simulink model "anti_windup_DC_motor_discrete"  (R2021a)
settings: Solver=VariableStepAuto  StartTime=0.0  StopTime=200  RelTol=1e-3
libraries: pid_lib x2
settings Model: Creator=kjartan  LastModifiedBy=kjartan

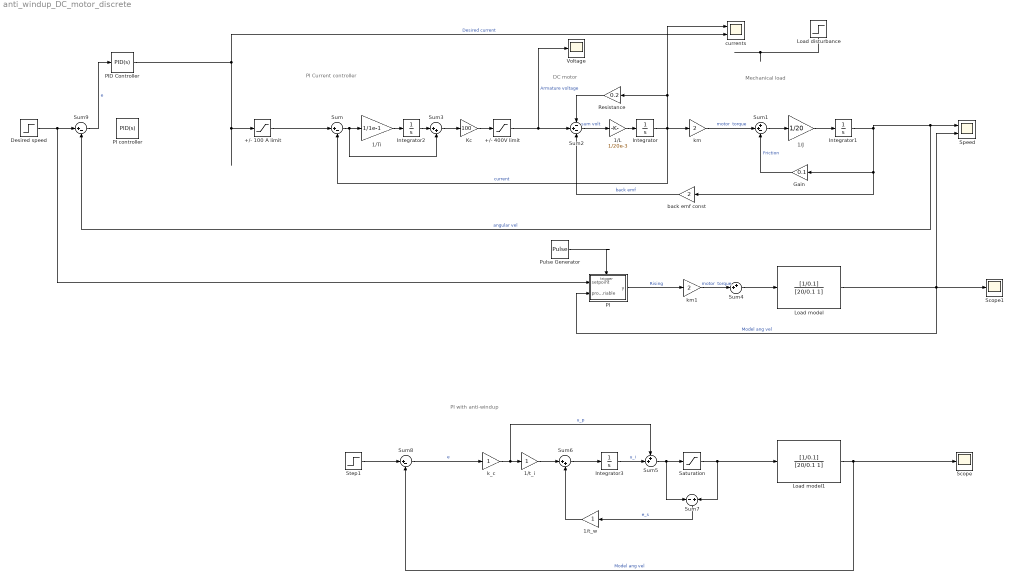
== system anti_windup_DC_motor_discrete ==
  note: PI with anti-windup
  note: PI Current controller
  note: Mechanical load
  note: DC motor
  +/- 100 A limit : Saturate  UpperLimit=100  LowerLimit=-100
  +/- 400V limit : Saturate  UpperLimit=400  LowerLimit=-400
  1/J : Gain  Gain=1/20
  1/L : Gain  Gain=1/20e-3
  1/Ti : Gain  Gain=1/1e-1
  1/t_i : Gain
  1/t_w : Gain
  Desired speed : Step  Time=0  After=100  SampleTime=0
  Gain : Gain  Gain=0.1
  Integrator{,1..3} (4 alike) : Integrator
  Kc : Gain  Gain=100
  Load disturbance : Step  Time=10  After=10  SampleTime=0
  Load model : TransferFcn  Numerator=[1/0.1]  Denominator=[20/0.1 1]
  Load model1 : TransferFcn  Numerator=[1/0.1]  Denominator=[20/0.1 1]
  PI : Subsystem
  PI controller : pid_lib/PID Controller  Controller=PID  Form=Ideal  TimeDomain=Continuous-time  UseExternalTs=off  SampleTime=-1  IntegratorMethod=Forward Euler  FilterMethod=Forward Euler  ControllerParametersSource=internal  P=10  I=1/20  D=20  UseFilter=on  N=100  TunerSelectOption=Transfer Function Based (PID Tuner App)  InitialConditionSource=internal  InitialConditionForIntegrator=0  InitialConditionForFilter=0  DifferentiatorICPrevScaledInput=0  ExternalReset=none  TrackingMode=off  Kt=1  LimitOutput=off  SatLimitsSource=internal  UpperSaturationLimit=inf  LowerSaturationLimit=-inf  LinearizeAsGain=on  AntiWindupMode=none  Kb=1  POutMin=[]  POutMax=[]  IOutMin=[]  IOutMax=[]  DOutMin=[]  DOutMax=[]  NOutMin=[]  NOutMax=[]  SumOutMin=[]  SumOutMax=[]  SaturationOutMin=[]  SaturationOutMax=[]  PParamMin=[]  PParamMax=[]  IParamMin=[]  IParamMax=[]  DParamMin=[]  DParamMax=[]  NParamMin=[]  NParamMax=[]  KbParamMin=[]  KbParamMax=[]  KtParamMin=[]  KtParamMax=[]  KbOutMin=[]  KbOutMax=[]  KtOutMin=[]  KtOutMax=[]  IntegratorOutMin=[]  IntegratorOutMax=[]  FilterOutMin=[]  FilterOutMax=[]  SumI1OutMin=[]  SumI1OutMax=[]  SumI2OutMin=[]  SumI2OutMax=[]  SumI3OutMin=[]  SumI3OutMax=[]  SumI4OutMin=[]  SumI4OutMax=[]  SumDOutMin=[]  SumDOutMax=[]  DifferentiatorOutMin=[]  DifferentiatorOutMax=[]  FilterDiffOutCoefMin=[]  FilterDiffOutCoefMax=[]  ReciprocalOutMin=[]  ReciprocalOutMax=[]  SumDenOutMin=[]  SumDenOutMax=[]  SumNumOutMin=[]  SumNumOutMax=[]  DivideOutMin=[]  DivideOutMax=[]  UdiffTsProdOutMin=[]  UdiffTsProdOutMax=[]  NTsProdOutMin=[]  NTsProdOutMax=[]  UintegralTsProdOutMin=[]  UintegralTsProdOutMax=[]  UngainTsProdOutMin=[]  UngainTsProdOutMax=[]  IntegratorContinuousStateAttributes=''  IntegratorStateMustResolveToSignalObject=off  IntegratorRTWStateStorageClass=Auto  FilterContinuousStateAttributes=''  FilterStateMustResolveToSignalObject=off  FilterRTWStateStorageClass=Auto  ParallelPVariant=Passthrough  IdealPVariant=InternalParameters  IVariant=InternalParameters  DVariant=InternalParameters  IntegratorVariant=Continuous  SatVariant=Disabled  AWVariant=Passthrough  PCopyVariant=Disabled  TRVariant=Disabled  FdbkBlocksVariant=Forward  IdealPFdbkVariant=Disabled  SatFdbkVariant=Disabled  DerivativeFilterVariant=ContFilter  NVariant=InternalParameters  NCopyVariant=Disabled  FilterICVariant=InternalICsFilter  IntegratorICVariant=InternalICs  ExternalResetVariant=Disabled  TRSumVariant=Passthrough  SumFdbkVariant=Disabled  SumVariant=Sum_PID  TsampFilterVariant=InternalTs  TsampNgainVariant=Passthrough  TsampIntegralVariant=Passthrough  ExternalSaturationOutDataTypeStr=Inherit: Same as second input
  PID Controller : pid_lib/PID Controller  Controller=PID  Form=Ideal  TimeDomain=Continuous-time  UseExternalTs=off  SampleTime=-1  IntegratorMethod=Forward Euler  FilterMethod=Forward Euler  ControllerParametersSource=internal  P=20  I=1/2  D=0  UseFilter=on  N=100  TunerSelectOption=Transfer Function Based (PID Tuner App)  InitialConditionSource=internal  InitialConditionForIntegrator=0  InitialConditionForFilter=0  DifferentiatorICPrevScaledInput=0  ExternalReset=none  TrackingMode=off  Kt=1  LimitOutput=off  SatLimitsSource=internal  UpperSaturationLimit=inf  LowerSaturationLimit=-inf  LinearizeAsGain=on  AntiWindupMode=none  Kb=1  POutMin=[]  POutMax=[]  IOutMin=[]  IOutMax=[]  DOutMin=[]  DOutMax=[]  NOutMin=[]  NOutMax=[]  SumOutMin=[]  SumOutMax=[]  SaturationOutMin=[]  SaturationOutMax=[]  PParamMin=[]  PParamMax=[]  IParamMin=[]  IParamMax=[]  DParamMin=[]  DParamMax=[]  NParamMin=[]  NParamMax=[]  KbParamMin=[]  KbParamMax=[]  KtParamMin=[]  KtParamMax=[]  KbOutMin=[]  KbOutMax=[]  KtOutMin=[]  KtOutMax=[]  IntegratorOutMin=[]  IntegratorOutMax=[]  FilterOutMin=[]  FilterOutMax=[]  SumI1OutMin=[]  SumI1OutMax=[]  SumI2OutMin=[]  SumI2OutMax=[]  SumI3OutMin=[]  SumI3OutMax=[]  SumI4OutMin=[]  SumI4OutMax=[]  SumDOutMin=[]  SumDOutMax=[]  DifferentiatorOutMin=[]  DifferentiatorOutMax=[]  FilterDiffOutCoefMin=[]  FilterDiffOutCoefMax=[]  ReciprocalOutMin=[]  ReciprocalOutMax=[]  SumDenOutMin=[]  SumDenOutMax=[]  SumNumOutMin=[]  SumNumOutMax=[]  DivideOutMin=[]  DivideOutMax=[]  UdiffTsProdOutMin=[]  UdiffTsProdOutMax=[]  NTsProdOutMin=[]  NTsProdOutMax=[]  UintegralTsProdOutMin=[]  UintegralTsProdOutMax=[]  UngainTsProdOutMin=[]  UngainTsProdOutMax=[]  IntegratorContinuousStateAttributes=''  IntegratorStateMustResolveToSignalObject=off  IntegratorRTWStateStorageClass=Auto  FilterContinuousStateAttributes=''  FilterStateMustResolveToSignalObject=off  FilterRTWStateStorageClass=Auto  ParallelPVariant=Passthrough  IdealPVariant=InternalParameters  IVariant=InternalParameters  DVariant=InternalParameters  IntegratorVariant=Continuous  SatVariant=Disabled  AWVariant=Passthrough  PCopyVariant=Disabled  TRVariant=Disabled  FdbkBlocksVariant=Forward  IdealPFdbkVariant=Disabled  SatFdbkVariant=Disabled  DerivativeFilterVariant=ContFilter  NVariant=InternalParameters  NCopyVariant=Disabled  FilterICVariant=InternalICsFilter  IntegratorICVariant=InternalICs  ExternalResetVariant=Disabled  TRSumVariant=Passthrough  SumFdbkVariant=Disabled  SumVariant=Sum_PID  TsampFilterVariant=InternalTs  TsampNgainVariant=Passthrough  TsampIntegralVariant=Passthrough  ExternalSaturationOutDataTypeStr=Inherit: Same as second input
  Pulse Generator : DiscretePulseGenerator  PulseType=Time based  Period=1e-2  PulseWidth=5
  Resistance : Gain  Gain=0.2
  Saturation : Saturate
  Scope : Scope
  Scope1 : Scope
  Speed : Scope  NumInputPorts=2
  Step1 : Step  After=100  SampleTime=0
  Sum : Sum  Inputs=|+-
  Sum1 : Sum  Inputs=++-
  Sum2 : Sum  Inputs=-+-
  Sum3 : Sum  Inputs=|++
  Sum4 : Sum  Inputs=++|
  Sum5 : Sum  Inputs=++|
  Sum6 : Sum  Inputs=|++
  Sum7 : Sum  Inputs=-|+
  Sum8 : Sum  Inputs=|+-
  Sum9 : Sum  Inputs=|+-
  Voltage : Scope
  back emf const : Gain  Gain=2
  currents : Scope  NumInputPorts=2
  k_c : Gain
  km : Gain  Gain=2
  km1 : Gain  Gain=2
  wires:
  Integrator1/1 -> back emf const/1, Gain/1, Sum9/2, Speed/1  "angular vel"
  1/L/1 -> Integrator/1
  Integrator/1 -> Sum/2, currents/1, Resistance/1, km/1  "current"
  km/1 -> Sum1/2  "motor  torque"
  Sum1/1 -> 1/J/1
  1/J/1 -> Integrator1/1
  Gain/1 -> Sum1/3  "Friction"
  Sum2/1 -> 1/L/1  "sum volt"
  back emf const/1 -> Sum2/3  "back emf"
  +/- 400V limit/1 -> Voltage/1, Sum2/2  "Armature voltage"
  Resistance/1 -> Sum2/1
  Kc/1 -> +/- 400V limit/1
  Sum3/1 -> Kc/1
  Integrator2/1 -> Sum3/1
  1/Ti/1 -> Integrator2/1
  Sum/1 -> Sum3/2, 1/Ti/1
  +/- 100 A limit/1 -> Sum/1
  PID Controller/1 -> +/- 100 A limit/1, currents/2  "Desired current"
  Load disturbance/1 -> ?
  Sum4/1 -> Load model/1
  Load model/1 -> PI/2(process variable), Scope1/1, Speed/2  "Model ang vel"
  Sum5/1 -> Sum7/1, Saturation/1
  Saturation/1 -> Sum7/2, Load model1/1
  Integrator3/1 -> Sum5/2  "u_i"
  Sum6/1 -> Integrator3/1
  1/t_w/1 -> Sum6/2
  Sum7/1 -> 1/t_w/1  "e_s"
  Sum8/1 -> k_c/1  "e"
  Load model1/1 -> Scope/1, Sum8/2  "Model ang vel"
  1/t_i/1 -> Sum6/1
  k_c/1 -> Sum5/1, 1/t_i/1  "u_p"
  Step1/1 -> Sum8/1
  km1/1 -> Sum4/2  "motor  torque"
  Sum9/1 -> PID Controller/1  "e"
  Desired speed/1 -> PI/1(setpoint), Sum9/1
  Pulse Generator/1 -> PI/Trigger
  PI/1(y) -> km1/1  "Rising"

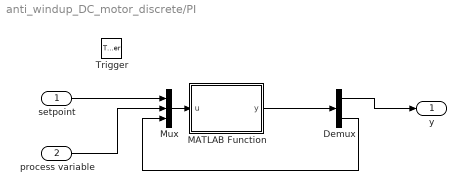
== system anti_windup_DC_motor_discrete/PI ==
  setpoint : Inport
  process variable : Inport  Port=2
  Trigger : TriggerPort  VariantControl=(inherit)
  Demux : Demux  Outputs=2
  MATLAB Function : MATLAB Function  TreatAsAtomicUnit=on
  Mux : Mux  Inputs=3
  y : Outport  InitialOutput=0  VectorParamsAs1DForOutWhenUnconnected=off
  wires:
  setpoint/1 -> Mux/1
  process variable/1 -> Mux/2
  Mux/1 -> MATLAB Function/1(u)
  MATLAB Function/1(y) -> Demux/1
  Demux/1 -> y/1
  Demux/2 -> Mux/3

== matlab function anti_windup_DC_motor_discrete/PI/MATLAB Function ==
  data: u input; y output
function y = PI_update(u)

% Anti-windup using backtracking

% Gains
kc = 10;
t_i = 2;
highlim = 100;
lowlim = -100;
h=0.01;

% Signals
sp = u(1); % Setpoint
pv = u(2); % process variable

uI = u(3); % Integral state

e = sp-pv; % Control error
v = kc*e + uI*kc/t_i;
if v > highlim
    y1 = highlim
    uI = uI - 1/t_i*(v-highlim);
elseif v < lowlim
    y1 = lowlim;
    uI = uI - 1/t_i*(v - lowlim);
else
    y1 = v;
    uI = uI + h*e;
end
y = [y1;uI];
